simulink model "MPC"  (R2021a)
settings: Solver=VariableStepAuto  StartTime=0.0  StopTime=10  RelTol=1e-3
values from neighbouring files (symbols this model uses):
  A = 0.14    [CarDynamics.m]    (also in LongDynWorking.m = 2.14; MPC_Script.m = [-(lf^2*Cf+lr^2*Cr)/(Iz*vx) (-lf*Cf+lr*Cr)/(Iz); MPC_Sim.m = [-(lf^2*Cf+lr^2*Cr)/(Iz*vx) (-lf*Cf+lr*Cr)/(Iz))
  B = 2*(2-mu)*8.3278    (= 24.9834)    [LongDynWorking.m]    (also in MPC_Script.m = [lf*Cf/Iz; Cf/(m*vx)]; MPC_Sim.m = [lf*Cf/Iz; Cf/(m*vx)])
  controller = optimizer(constraints, objective,[],{x{1},r,Ad_,Bd_},[u{:}])    [MPC_Script.m]
  Ts = 0.01    [MPC_Script.m]    (also in MPC_Sim.m)
undefined symbols (not defined in the file or in its folder): LongDynWorking, MPC_Sim
settings Model: Creator=bensalso  LastModifiedBy=21655
settings SolverCC: AlgebraicLoopSolver=TrustRegion
settings DataIOCC: ReturnWorkspaceOutputs=off
settings DebuggingCC: SFMachineParentedDataDiag=warning  ArithmeticOperatorsInVariantConditions=warning
settings SFSimCC: CustomCodeUndefinedFunction=UseInterfaceOnly

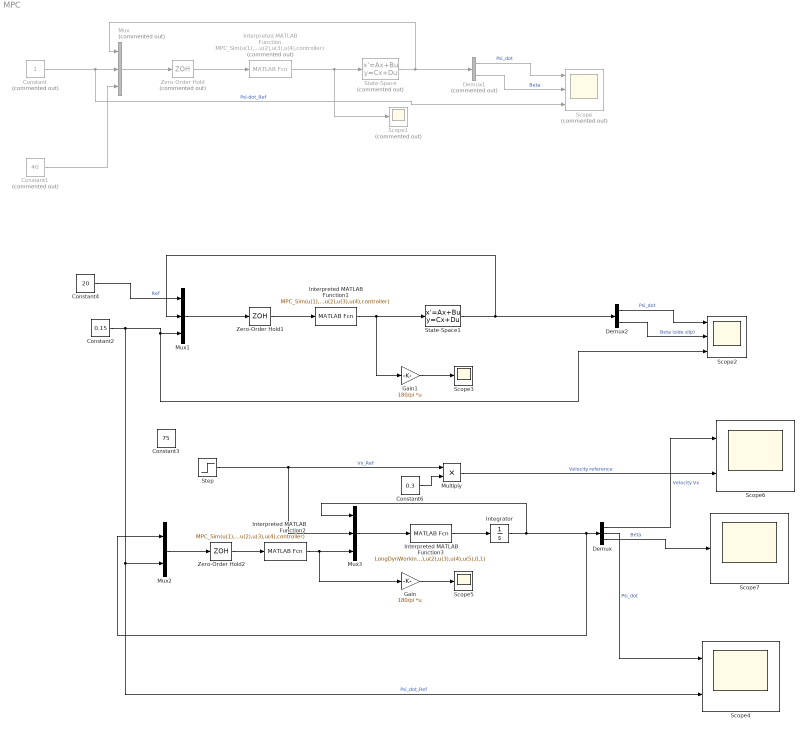
== system MPC ==
  Constant : Constant  Commented=on
  Constant1 : Constant  Commented=on  Value=40
  Constant2 : Constant  Value=0.15
  Constant3 : Constant  Value=75
  Constant4 : Constant  Value=20
  Constant6 : Constant  Value=0.3
  Demux : Demux  Outputs=3
  Demux1 : Demux  Commented=on  Outputs=2
  Demux2 : Demux  Outputs=2
  Gain : Gain  Gain=180/pi  Multiplication=Matrix(K*u) (u vector)
  Gain1 : Gain  Gain=180/pi  Multiplication=Matrix(K*u) (u vector)
  Integrator : Integrator  InitialCondition=[20 ; 0 ; 0]
  Interpreted MATLAB Function : MATLABFcn  Commented=on  MATLABFcn=MPC_Sim(u(1),u(2),u(3),u(4),controller)  OutputDimensions=1
  Interpreted MATLAB Function1 : MATLABFcn  MATLABFcn=MPC_Sim(u(1),u(2),u(3),u(4),controller)  OutputDimensions=1
  Interpreted MATLAB Function2 : MATLABFcn  MATLABFcn=MPC_Sim(u(1),u(2),u(3),u(4),controller)  OutputDimensions=1
  Interpreted MATLAB Function3 : MATLABFcn  MATLABFcn=LongDynWorking(u(1),u(2),u(3),u(4),u(5),0,1)  OutputDimensions=3
  Multiply : Product
  Mux : Mux  Commented=on  Inputs=3
  Mux1 : Mux  Inputs=3
  Mux2 : Mux  Inputs=2
  Mux3 : Mux  Inputs=3
  Scope : Scope  Commented=on  NumInputPorts=3
  Scope1 : Scope  Commented=on
  Scope2 : Scope  NumInputPorts=3
  Scope3 : Scope
  Scope4 : Scope  NumInputPorts=2
  Scope5 : Scope
  Scope6 : Scope  NumInputPorts=2
  Scope7 : Scope
  State-Space : StateSpace  Commented=on  A=A  B=B  C=eye(2)  D=[0;0]  InitialCondition=0
  State-Space1 : StateSpace  A=A  B=B  C=eye(2)  D=[0;0]  InitialCondition=0
  Step : Step  Time=5  Before=75  After=50  SampleTime=0
  Zero-Order Hold : ZeroOrderHold  Commented=on  SampleTime=Ts
  Zero-Order Hold1 : ZeroOrderHold  SampleTime=Ts
  Zero-Order Hold2 : ZeroOrderHold  SampleTime=Ts
  wires:
  State-Space/1 -> Demux1/1, Mux/1
  Interpreted MATLAB Function/1 -> Scope1/1, State-Space/1
  Zero-Order Hold/1 -> Interpreted MATLAB Function/1
  Mux/1 -> Zero-Order Hold/1
  Constant/1 -> Scope/3, Mux/2  "Psi-dot_Ref"
  Constant1/1 -> Mux/3
  Constant2/1 -> Scope4/2, Mux2/2, Scope2/3, Mux1/3  "Psi_dot_Ref"
  Mux1/1 -> Zero-Order Hold1/1
  State-Space1/1 -> Demux2/1, Mux1/2
  Zero-Order Hold1/1 -> Interpreted MATLAB Function1/1
  Interpreted MATLAB Function1/1 -> Gain1/1, State-Space1/1
  Zero-Order Hold2/1 -> Interpreted MATLAB Function2/1
  Interpreted MATLAB Function3/1 -> Integrator/1
  Mux2/1 -> Zero-Order Hold2/1
  Gain/1 -> Scope5/1
  Integrator/1 -> Mux3/1, Mux2/1, Demux/1
  Interpreted MATLAB Function2/1 -> Gain/1, Mux3/3
  Step/1 -> Multiply/1, Mux3/2  "Vx_Ref"
  Mux3/1 -> Interpreted MATLAB Function3/1
  Gain1/1 -> Scope3/1
  Constant4/1 -> Mux1/1  "Ref"
  Demux1/2 -> Scope/2  "Beta"
  Demux1/1 -> Scope/1  "Psi_dot"
  Demux/2 -> Scope4/1  "Psi_dot"
  Demux2/1 -> Scope2/1  "Psi_dot"
  Demux2/2 -> Scope2/2  "Beta (side slip)"
  Demux/1 -> Scope6/1  "Velocity Vx"
  Demux/3 -> Scope7/1  "Beta"
  Multiply/1 -> Scope6/2  "Velocity reference"
  Constant6/1 -> Multiply/2
